simulink model "robotarm_student_2021a_Ebox"  (R2024a)
settings: Solver=FixedStepDiscrete  StartTime=0.0  StopTime=tsim  FixedStep=Ts  RelTol=1e-3  EnableMultiTasking=on
InitFcn:
  | Fs = 2048; Ts = 1/Fs;tsim = inf;
undefined symbols (not defined in the file or in its folder): DiscIntNeverNeededParam
libraries: sperte_lib x29, simulink x5, raspberrypiCommlib x2
(part 2 of 2)

== system robotarm_student_2021a_Ebox/RobotArm/Supervisor/Subsystem/LED Ring/Subsystem3/If Action Subsystem1 ==
  In1 : Inport
  Action Port : ActionPort  ActionPortLabel=else
  Constant : Constant  Value=13  OutDataTypeStr=uint8
  Matrix Concatenate : Concatenate  ConcatenateDimension=2
  Serial Write : raspberrypiCommlib/Serial Write  board=Pi 4 Model B  SCIModule_=/dev/ttyACM0  Baudrate_=9600  Parity=None  StopBits_=1  HardwareFlowControl=None  ByteOrder=LittleEndian  OutputStatus=off  blockPlatform=RaspberryPi
  String Concatenate : StringConcatenate
  String Constant3 : StringConstant  String='color '
  String to ASCII : StringToASCII
  wires:
  Matrix Concatenate/1 -> Serial Write/1
  String to ASCII/1 -> Matrix Concatenate/1
  String Concatenate/1 -> String to ASCII/1
  String Constant3/1 -> String Concatenate/1
  Constant/1 -> Matrix Concatenate/2
  In1/1 -> String Concatenate/2

== matlab function robotarm_student_2021a_Ebox/RobotArm/Supervisor/Supervisory Controller R/Angle2Z ==
  data: u input; y output
function y = fcn(u)

% Z and X angles to height of the robotarm. The initial angles are the
% angles from the horizontal line to the correponding arm.

initialanglez = 0.6150;
initialanglex = (75.3841/180)*pi;
thetax = -u(2)+initialanglex;
thetaz = u(3)+initialanglez;

theta1 = thetax;
theta2 = thetaz;

% parameters

l1 = 80e-3;
l2 = 130e-3;
l3 = 165e-3;
l4 = 130e-3;
l5 = 120e-3;
l6 = 120e-3 + 65e-3;
length_head = 45e-3;
l7 = 81e-3;

% functions

fx1 = l1*cos(theta1);
fy1 = l1*sin(theta1);

fx2 = l2*cos(theta2);
fy2 = l3 + l2*sin(theta2);

d12 = sqrt((fx2 - fx1)^2 + (fy2 - fy1)^2);
d13 = sqrt(fx1^2 + (l3 - fy1)^2);

phi1 = acos((l2^2 + d12^2 -d13^2)/(2*d12*l2));
phi2 = acos((l5^2 + d12^2 -l4^2)/(2*d12*l5));

yf = fy2- l6*sin(pi - phi1 - phi2 - theta2);

y = yf-length_head+l7;

== matlab function robotarm_student_2021a_Ebox/RobotArm/Supervisor/Supervisory Controller Z/Angle2Z ==
  data: u input; y output
function y = fcn(u)

% Z and X angles to height of the robotarm. The initial angles are the
% angles from the horizontal line to the correponding arm.

initialanglez = 0.6150;
initialanglex = (75.3841/180)*pi;
thetax = -u(2)+initialanglex;
thetaz = u(3)+initialanglez;

theta1 = thetax;
theta2 = thetaz;

% parameters

l1 = 80e-3;
l2 = 130e-3;
l3 = 165e-3;
l4 = 130e-3;
l5 = 120e-3;
l6 = 120e-3 + 65e-3;
length_head = 45e-3;
l7 = 81e-3;

% functions

fx1 = l1*cos(theta1);
fy1 = l1*sin(theta1);

fx2 = l2*cos(theta2);
fy2 = l3 + l2*sin(theta2);

d12 = sqrt((fx2 - fx1)^2 + (fy2 - fy1)^2);
d13 = sqrt(fx1^2 + (l3 - fy1)^2);

phi1 = acos((l2^2 + d12^2 -d13^2)/(2*d12*l2));
phi2 = acos((l5^2 + d12^2 -l4^2)/(2*d12*l5));

yf = fy2- l6*sin(pi - phi1 - phi2 - theta2);

y = yf-length_head+l7;

== stateflow chart robotarm_student_2021a_Ebox/Controller/Stateflow  ==
  settings: executeAtInitialization=1
  state Object_Detection [parallel]
    settings: executionOrder=1
    state Seeking
      entry:
    state WaitSeeking
      entry:
      GetProduct
    (default) -> Seeking
    (junction 9) -> Seeking
    (junction 7) -> (junction 9)
    Seeking -> WaitSeeking : [nObject>=1]
    WaitSeeking -> (junction 7) : ScanAgain
  state Belt [parallel]
    settings: executionOrder=2
    state Belt_Home
      during:
      Conveyor = -20;
    (default) -> Belt_Home
  state Robot_Arm [parallel]
    settings: executionOrder=3
    state Start_Home
      entry:
      R_rad = 0;
      X_rad = 0;
      Z_rad = 0;
    state Move_XY
      entry:
      VacuumOn
      R_rad = atan(Y_in/X_in);
      X_rad = 0;
      Z_rad = 0;
    (default) -> Start_Home
    Start_Home -> Move_XY : GetProduct
  state Vacuum [parallel]
    settings: executionOrder=4
    state Vacuum_Off
      during:
      Pump = 0;
      Blow_suck = 0
    (default) -> Vacuum_Off
  data: X_in input; Y_in input; nObject input; VacuumSensor input; R_rad output; X_rad output; Z_rad output; Pump output; Blow_suck output; Conveyor output
  events: VacuumOn local FUNCTION_CALL_EVENT; Release local FUNCTION_CALL_EVENT; GetProduct local FUNCTION_CALL_EVENT; ScanAgain local FUNCTION_CALL_EVENT; ObjectProduct local FUNCTION_CALL_EVENT; Gripped local FUNCTION_CALL_EVENT; GoHome local FUNCTION_CALL_EVENT

== stateflow chart robotarm_student_2021a_Ebox/RobotArm/Supervisor/Supervisory Conveyor/Supervisor ==
  state Waiting
    %Homing has to wait for 3 sec
    %as the new arm gets the 5V enable signal
    %after pressing start to avoi d moving to X0 too
    %early
  state Homing
    entry:
    %Set jog speed and homing state
    Ready=0;
    homingBusy = 1;
    jogSpeed = 20;
    homeControllerEnabled=1;
  state MovetoX0
    entry:
    jogSpeed = -20;
  state CheckRobotIsON
    entry:
    jogSpeed = 0;
  state WaitForRest
    entry: Ready = 1;
  state EnableRunAndSafety
    entry:
    resetEnc=0;
    homingBusy=0;
  state ResetEnc
    entry:
    resetEnc=1;
    homeControllerEnabled=0;
  (default) -> Waiting
  Waiting -> Homing : after(1,sec)
  Homing -> MovetoX0 : after(3,sec)
  MovetoX0 -> CheckRobotIsON : %Allow time for moving
      | after(3,sec)
  CheckRobotIsON -> WaitForRest : after(1,sec)
  WaitForRest -> ResetEnc : [AllReady]
  ResetEnc -> EnableRunAndSafety : after(1,sec)
  data: jogSpeed output double; homeControllerEnabled output double; resetEnc output double; homingBusy output double =1; Ready output double =1; AllReady input boolean; StopSim output double =0

== stateflow chart robotarm_student_2021a_Ebox/RobotArm/Supervisor/Supervisory Controller R/Supervisor ==
  state Waiting
    %Homing has to wait for 3 sec
    %as the new arm gets the 5V enable signal
    %after pressing start to avoid moving to X0 too
    %early
    Ready=0;
    toPoint = 0;
    homingBusy = 1;
    jogSpeed = -0.001;
    homeControllerEnabled=0.01;
  state Waiting1
    %Homing has to wait for 3 sec
    %as the new arm gets the 5V enable signal
    %after pressing start to avoid moving to X0 too
    %early
    Ready=0;
    toPoint = 0;
    homingBusy = 1;
    jogSpeed = 0;
    homeControllerEnabled=1;
  state AirbagLeft
    entry:
    homingBusy = 1;
    currentcarPos = carPos;
    airBagEnabled = 1;
    airBagRef=currentcarPos+0.02;
  state DisableOutputs
    entry:
    controlEnabled=0;
    StopSim = 1;
  state Homing
    entry:
    %Set jog speed and homing state
    Ready=0;
    toPoint = 0;
    homingBusy = 1;
    jogSpeed = -0.4;
    homeControllerEnabled=1;
  state AirbagLeft1
    entry:
    homingBusy = 1;
    currentcarPos = carPos;
    airBagEnabled = 1;
    airBagRef=currentcarPos-0.02;
  state AirbagConveyor
    entry:
    homingBusy = 1;
    currentcarPos = carPos;
    airBagEnabled = 1;
    airBagRef=currentcarPos+0.02
  state MovetoX0
    entry:
    jogSpeed = 0.0;
    toPoint = Offset_homing
  state STOPRobotIsOFF
    entry:
    StopSim=1;
  state CheckRobotIsON
  state EnableRunAndSafety
    entry:
    resetEnc=0;
    homingBusy=0;
  state RobotIsON
  state WaitForRest
    entry: Ready = 1;
  state ResetEnc
    entry:
    homingBusy = 100;
    resetEnc=1;
    homeControllerEnabled=0;
  (default) -> Waiting
  Waiting -> Waiting1 : after(1,sec)
  Waiting1 -> Homing : after(3,sec)
  AirbagLeft -> DisableOutputs : after(3,sec)
  AirbagConveyor -> DisableOutputs : after(3,sec)
  AirbagLeft1 -> DisableOutputs : after(3,sec)
  EnableRunAndSafety -> AirbagLeft [order 2] : [carPos<-1.1]
  Homing -> MovetoX0 : %Transition if homeswitch becomes high
      | [homeSwitch]
  EnableRunAndSafety -> AirbagLeft1 [order 1] : [carPos>2.7]
  EnableRunAndSafety -> AirbagConveyor [order 3] : [zcoordinate<0.056&&carPos < 1.3]
  MovetoX0 -> CheckRobotIsON [order 2] : % Allow time for moving
      | after(5,sec)
  MovetoX0 -> CheckRobotIsON [order 1] : [carPos == toPoint]
  CheckRobotIsON -> STOPRobotIsOFF [order 1] : [carPos<-3]
  CheckRobotIsON -> RobotIsON [order 2]
  RobotIsON -> WaitForRest : after(1,sec)
  ResetEnc -> EnableRunAndSafety : after(1,sec)
  WaitForRest -> ResetEnc : [AllReady]
  data: jogSpeed output double; toPoint output double; homeControllerEnabled output double; resetEnc output double; homingBusy output double =1; homeSwitch input boolean; carPos input double; airBagEnabled output double =0; airBagRef output double =0; controlEnabled output double =1; Ready output double =1; AllReady input boolean; StopSim output double =0; zcoordinate input; currentcarPos local double; Offset_homing input

== stateflow chart robotarm_student_2021a_Ebox/RobotArm/Supervisor/Supervisory Controller X/Supervisor ==
  state Waiting
    %Homing has to wait for 3 sec
    %as the new arm gets the 5V enable signal
    %after pressing start to avoid moving to X0 too
    %early
    Ready=0;
    toPoint = 0;
    homingBusy = 1;
    jogSpeed = -0.001;
    homeControllerEnabled=0.01;
  state DisableOutputs
    entry:
    controlEnabled=0;
    StopSim=1;
  state AirbagLeft
    entry:
    homingBusy = 1;
    currentcarPos = carPos;
    airBagEnabled = 1;
    airBagRef=currentcarPos+0.02;
  state Waiting1
    %Homing has to wait for 3 sec
    %as the new arm gets the 5V enable signal
    %after pressing start to avoid moving to X0 too
    %early
    Ready=0;
    toPoint = 0;
    homingBusy = 1;
    jogSpeed = 0;
    homeControllerEnabled=1;
  state AirbagRight
    entry:
    homingBusy = 1;
    currentcarPos = carPos;
    airBagEnabled = 1;
    airBagRef=currentcarPos-0.02;
  state Homing
    entry:
    %Set jog speed and homing state
    jogSpeed = -0.2;
    homeControllerEnabled=1;
  state MovetoX0
    entry:
    jogSpeed = 0.0;
    toPoint = offset_homing;
  state EnableRunAndSafety
    entry:
    resetEnc=0;
    homingBusy=0;
  state WaitForRest
    entry: Ready = 1;
  state ResetEnc
    entry:
    resetEnc=1;
    homeControllerEnabled=0;
  (default) -> Waiting
  Waiting -> Waiting1 : after(2,sec)
  AirbagLeft -> DisableOutputs : after(3,sec)
  AirbagRight -> DisableOutputs : after(3,sec)
  EnableRunAndSafety -> AirbagLeft [order 1] : [carPos<-0.5]
  Waiting1 -> Homing : after(3,sec)
  EnableRunAndSafety -> AirbagRight [order 2] : [carPos>1.1 ]
  Homing -> MovetoX0 : %Transition if homeswitch becomes high
      | [homeSwitch]
  MovetoX0 -> WaitForRest [order 2] : %Allow time for moving
      | after(5,sec)
  MovetoX0 -> WaitForRest [order 1] : [carPos == toPoint]
  ResetEnc -> EnableRunAndSafety : after(1,sec)
  WaitForRest -> ResetEnc : [AllReady]
  data: jogSpeed output double; toPoint output double; homeControllerEnabled output double; resetEnc output double; homingBusy output double =1; homeSwitch input boolean; carPos input double; airBagEnabled output double =0; airBagRef output double =0; controlEnabled output double =1; Ready output double =1; AllReady input boolean; StopSim output double =0; currentcarPos local double; offset_homing input

== stateflow chart robotarm_student_2021a_Ebox/RobotArm/Supervisor/Supervisory Controller Z/Supervisor ==
  state Waiting
    %Homing has to wait for 3 sec
    %as the new arm gets the 5V enable signal
    %after pressing start to avoid moving to X0 too
    %early
    Ready=0;
    toPoint = 0;
    homingBusy = 1;
    jogSpeed = 0.001;
    homeControllerEnabled=0.1;
  state Waiting1
    %Homing has to wait for 3 sec
    %as the new arm gets the 5V enable signal
    %after pressing start to avoid moving to X0 too
    %early
    Ready=0;
    toPoint = 0;
    jogSpeed =  0 ;
    homeControllerEnabled=1;
  state DisableOutputs
    entry:
    controlEnabled=0;
    StopSim=1;
  state Homing
    entry:
    %Set jog speed and homing state
    toPoint = 0;
    Ready = 0;
    homingBusy = 1;
    jogSpeed = 0.2;
    homeControllerEnabled=1;
  state AirbagConveyor
    entry:
    homingBusy = 1;
    currentcarPos = carPos;
    airBagEnabled = 1;
    airBagRef=currentcarPos+0.1
  state MovetoX0
    entry:
    jogSpeed = 0.0;
    toPoint = offset_homing;
  state AirbagTop
    entry:
    homingBusy = 1;
    currentcarPos = carPos;
    airBagEnabled = 1;
    airBagRef=currentcarPos-0.02;
  state WaitForRest
    entry: Ready = 1;
  state EnableRunAndSafety
    entry:
    resetEnc=0;
    homingBusy=0;
  state AirbagDrop
    entry:
    homingBusy = 1;
    currentcarPos = carPos;
    airBagEnabled = 1;
    airBagRef=currentcarPos+0.02
  state ResetEnc
    entry:
    resetEnc=1;
    homeControllerEnabled=0;
    Ready = 1;
  (default) -> Waiting
  Waiting -> Waiting1 : after(2,sec)
  Waiting1 -> Homing : after(2,sec)
  AirbagDrop -> DisableOutputs : after(3,sec)
  AirbagConveyor -> DisableOutputs : after(3,sec)
  AirbagTop -> DisableOutputs : after(3,sec)
  EnableRunAndSafety -> AirbagConveyor [order 1] : [zcoordinate<0.056&&rcoordinate < 1.3]
  Homing -> MovetoX0 : %Transition if homeswitch becomes high
      | [homeSwitch]
  EnableRunAndSafety -> AirbagTop [order 2] : [carPos>0.3]
  MovetoX0 -> WaitForRest [order 2] : %Allow time for moving
      | after(5,sec)
  MovetoX0 -> WaitForRest [order 1] : [carPos == toPoint]
  WaitForRest -> ResetEnc : [AllReady]
  EnableRunAndSafety -> AirbagDrop [order 3] : [zcoordinate<0&&rcoordinate>1.3]
  ResetEnc -> EnableRunAndSafety : after(1,sec)
  data: jogSpeed output double; toPoint output double; homeControllerEnabled output double; resetEnc output double; homingBusy output double =1; homeSwitch input boolean; carPos input double; airBagEnabled output double =0; airBagRef output double =0; controlEnabled output double =1; Ready output double =1; AllReady input boolean; StopSim output double =0; zcoordinate input double; currentcarPos local double; rcoordinate input double; offset_homing input
